simulink model "rician_channel_rectangular"  (R2016b)
settings: Solver=FixedStepAuto  StartTime=0.0  StopTime=2e-6  FixedStep=2*10^(-11)  RelTol=1e-3  EnableMultiTasking=on
libraries: simulink x2, commchan3 x2
settings Model: Creator=MOMENT OF PEACE  LastModifiedBy=MOMENT OF PEACE
settings DataIOCC: LimitDataPoints=on  SaveFormat=Array
settings OptimizationCC: LifeSpan=inf
settings DebuggingCC: SFUnexpectedBacktrackingDiag=warning  SFNoUnconditionalDefaultTransitionDiag=warning  SFExecutionAtInitializationDiag=none
settings HardwareCC: ProdBitPerPointer=32  ProdBitPerSizeT=32  ProdBitPerPtrDiffT=32  ProdLargestAtomicFloat=None  ProdIntDivRoundTo=Undefined  ProdEndianess=Unspecified  ProdWordSize=32  ProdHWDeviceType=32-bit Generic
settings ModelReferenceCC: PropagateSignalLabelsOutOfModel=off
settings GRTTargetCC: TargetLangStandard=C89/C90 (ANSI)  GeneratePreprocessorConditionals=Disable all
settings ConfigComp: CovMetricSettings=dw  CovHtmlReporting=on  CovSaveCumulativeToWorkspaceVar=on  CovSaveSingleToWorkspaceVar=on  CovExternalEMLEnable=off

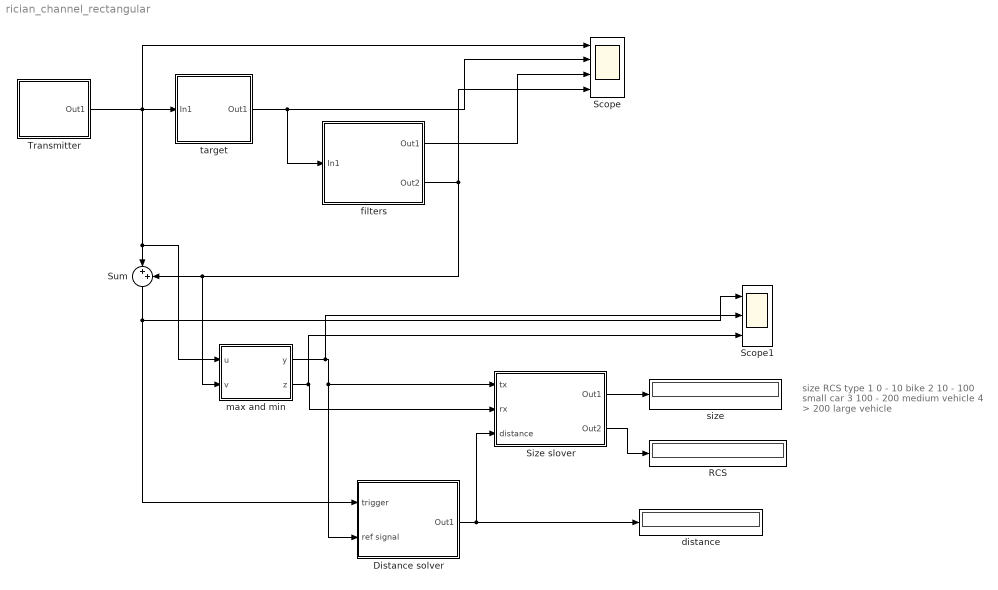
== system rician_channel_rectangular ==
  note: size RCS type
      | 1 0 - 10 bike
      | 2 10 - 100 small car
      | 3 100 - 200 medium vehicle
      | 4 > 200 large vehicle
  Distance solver : Subsystem
  RCS : Display
  Scope : Scope  NumInputPorts=4
  Scope1 : Scope  NumInputPorts=3
  Size slover : Subsystem
  Sum : Sum  Inputs=|++
  Transmitter : Subsystem
  distance : Display
  filters : Subsystem
  max and min : MATLAB Function  TreatAsAtomicUnit=on
  size : Display
  target : Subsystem  mask{d=15, v=30, s=150, snr=5, gain=10}
      mask prompts: d "Distance (m)"; v "Velocity (m/s)"; s "RCS (m^2)"; snr "SNR (dB)"; gain "Gain (dB)"
      mask init:
      | % d denotes the distance and v denotes velocity
      | c = 3e8;    % the speed of light
      | p = 1e-9;   % the width of impulse
      | r = 0.7;    % relectivity
      | rcs = s;
      | w = p * c;
      | 
      | G = 10^(gain/10);       % gain in decimal
      | delay = 2 * d / c;      % phase delay
      | loss = G^2 *  w^2 * rcs/((4 * pi)^3 * d^4);     % path loss
  wires:
  target/1(Out1) -> Scope/2, filters/1(In1)
  filters/1(Out1) -> Scope/3
  filters/2(Out2) -> max and min/2(v), Sum/2, Scope/4
  max and min/2(z) -> Scope1/3, Size slover/2(rx)
  Size slover/1(Out1) -> size/1
  Sum/1 -> Distance solver/1(trigger), Scope1/1
  Distance solver/1(Out1) -> distance/1, Size slover/3(distance)
  Transmitter/1(Out1) -> Scope/1, target/1(In1), max and min/1(u), Sum/1
  Size slover/2(Out2) -> RCS/1
  max and min/1(y) -> Scope1/2, Size slover/1(tx), Distance solver/2(ref signal)

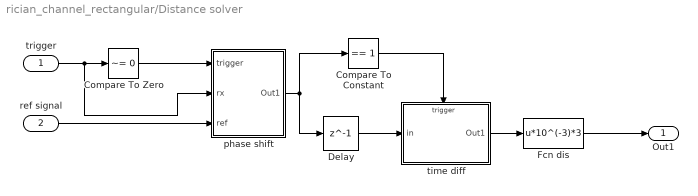
== system rician_channel_rectangular/Distance solver ==
  trigger : Inport
  ref signal : Inport  Port=2
  Compare To Constant : simulink/Logic and Bit Operations/Compare To Constant  relop===  const=1  OutDataTypeStr=boolean
  Compare To Zero : simulink/Logic and Bit Operations/Compare To Zero  relop=~=  OutDataTypeStr=uint8
  Delay : Delay  DelayLength=1  InitialCondition=0
  Fcn dis : Fcn  Expr=u*10^(-3)*3
  phase shift : Subsystem
  time diff : Subsystem  TreatAsAtomicUnit=on
  Out1 : Outport
  wires:
  ref signal/1 -> phase shift/3(ref)
  Fcn dis/1 -> Out1/1
  Compare To Constant/1 -> time diff/Trigger
  trigger/1 -> phase shift/2(rx), Compare To Zero/1
  time diff/1(Out1) -> Fcn dis/1
  Delay/1 -> time diff/1(in)
  phase shift/1(Out1) -> Compare To Constant/1, Delay/1
  Compare To Zero/1 -> phase shift/1(trigger)

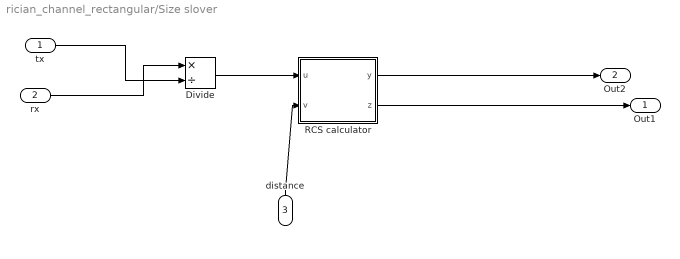
== system rician_channel_rectangular/Size slover ==
  tx : Inport
  rx : Inport  Port=2
  distance : Inport  Port=3
  Divide : Product  Inputs=*/
  RCS calculator : MATLAB Function  TreatAsAtomicUnit=on
  Out1 : Outport
  Out2 : Outport  Port=2
  wires:
  distance/1 -> RCS calculator/2(v)
  tx/1 -> Divide/2
  rx/1 -> Divide/1
  Divide/1 -> RCS calculator/1(u)
  RCS calculator/1(y) -> Out2/1
  RCS calculator/2(z) -> Out1/1

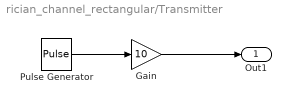
== system rician_channel_rectangular/Transmitter ==
  Gain : Gain  Gain=10
  Pulse Generator : DiscretePulseGenerator  Amplitude=0.004  Period=10000  PulseWidth=50  SampleTime=2e-11
  Out1 : Outport
  wires:
  Gain/1 -> Out1/1
  Pulse Generator/1 -> Gain/1

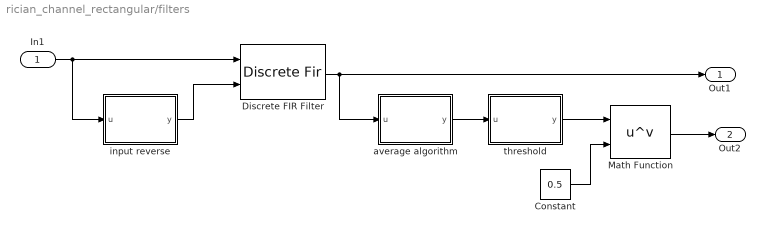
== system rician_channel_rectangular/filters ==
  In1 : Inport
  Constant : Constant  Value=0.5
  Discrete FIR Filter : DiscreteFir  CoefSource=Input port  Coefficients=[1 1 1 1 1 1]  InputProcessing=Columns as channels (frame based)
      settings: InputPortMap=u0,u1
  Math Function : Math  Operator=pow  SaturateOnIntegerOverflow=on
  average algorithm : MATLAB Function  TreatAsAtomicUnit=on
  input reverse : MATLAB Function  TreatAsAtomicUnit=on
  threshold : MATLAB Function  TreatAsAtomicUnit=on
  Out1 : Outport
  Out2 : Outport  Port=2
  wires:
  In1/1 -> Discrete FIR Filter/1, input reverse/1(u)
  average algorithm/1(y) -> threshold/1(u)
  Discrete FIR Filter/1 -> Out1/1, average algorithm/1(u)
  input reverse/1(y) -> Discrete FIR Filter/2
  threshold/1(y) -> Math Function/1
  Math Function/1 -> Out2/1
  Constant/1 -> Math Function/2

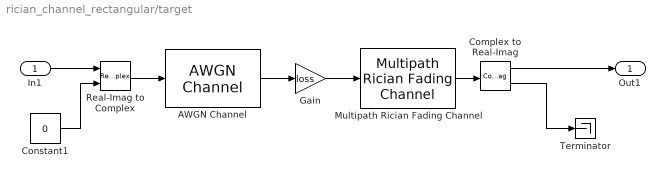
== system rician_channel_rectangular/target ==
  In1 : Inport
  AWGN Channel : commchan3/AWGN Channel  InputProcessing=Columns as channels (frame based)  seed=67  noiseMode="Signal to noise ratio  (SNR)"  EbNodB=10  EsNodB=10  SNRdB=snr  bitsPerSym=1  Ps=0.004/300  Tsym=1  variance=1
  Complex to Real-Imag : ComplexToRealImag
  Constant1 : Constant  Value=0
  Gain : Gain  Gain=loss
  Multipath Rician Fading Channel : commchan3/Multipath Rician Fading Channel  K=100  fdLOS=0  thetaLOS=0  maxDopplerShift=40  spectrumType=Jakes  sigmaGaussian=1/sqrt(2)  coeffRounded=[1 -1.72 0.785]  freqMinMaxRJakes=[0 1]  freqMinMaxAJakes=[0 1]  sigmaGaussian1=1/sqrt(2)  sigmaGaussian2=1/sqrt(2)  centerFreqGaussian1=0  centerFreqGaussian2=0  gainGaussian1=0.5  gainGaussian2=0.5  coeffBell=9  dopplerSpectrum=doppler.jakes  pathDelays=[delay delay+(5e-8) delay+(1e-7)]  avgPathGaindB=[0 -1 -1]  normalizePathGains=on  seed=73  enableProbe=0  openVisAtStart=off  outPathGains=off  outDelay=off
  Real-Imag to Complex : RealImagToComplex
  Terminator : Terminator
  Out1 : Outport
  wires:
  Complex to Real-Imag/1 -> Out1/1
  AWGN Channel/1 -> Gain/1
  Multipath Rician Fading Channel/1 -> Complex to Real-Imag/1
  Constant1/1 -> Real-Imag to Complex/2
  In1/1 -> Real-Imag to Complex/1
  Complex to Real-Imag/2 -> Terminator/1
  Real-Imag to Complex/1 -> AWGN Channel/1
  Gain/1 -> Multipath Rician Fading Channel/1

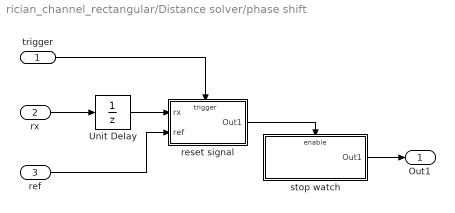
== system rician_channel_rectangular/Distance solver/phase shift ==
  trigger : Inport
  rx : Inport  Port=2
  ref : Inport  Port=3
  Unit Delay : UnitDelay  SampleTime=-1
  reset signal : Subsystem  TreatAsAtomicUnit=on
  stop watch : Subsystem  TreatAsAtomicUnit=on
  Out1 : Outport
  wires:
  reset signal/1(Out1) -> stop watch/Enable
  trigger/1 -> reset signal/Trigger
  stop watch/1(Out1) -> Out1/1
  rx/1 -> Unit Delay/1
  ref/1 -> reset signal/2(ref)
  Unit Delay/1 -> reset signal/1(rx)

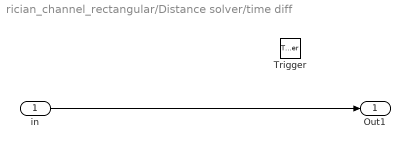
== system rician_channel_rectangular/Distance solver/time diff ==
  in : Inport
  Trigger : TriggerPort  VariantControl=Variant  ZeroCross=off
  Out1 : Outport
  wires:
  in/1 -> Out1/1

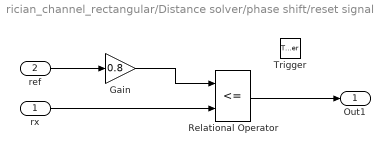
== system rician_channel_rectangular/Distance solver/phase shift/reset signal ==
  rx : Inport
  ref : Inport  Port=2
  Trigger : TriggerPort  TriggerType=falling  VariantControl=Variant
  Gain : Gain  Gain=0.8
  Relational Operator : RelationalOperator  Operator=<=  OutDataTypeStr=boolean  RndMeth=Nearest
  Out1 : Outport
  wires:
  ref/1 -> Gain/1
  Gain/1 -> Relational Operator/1
  rx/1 -> Relational Operator/2
  Relational Operator/1 -> Out1/1

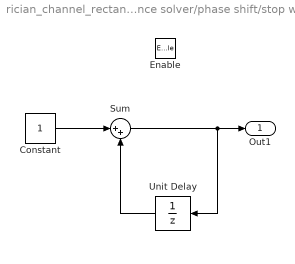
== system rician_channel_rectangular/Distance solver/phase shift/stop watch ==
  Enable : EnablePort  StatesWhenEnabling=reset
  Constant : Constant
  Sum : Sum  Inputs=|++
  Unit Delay : UnitDelay  SampleTime=-1
  Out1 : Outport
  wires:
  Constant/1 -> Sum/1
  Sum/1 -> Unit Delay/1, Out1/1
  Unit Delay/1 -> Sum/2

== matlab function rician_channel_rectangular/filters/average algorithm ==
  data: u input; y output
function y = fcn(u)
%#codegen
persistent summ;
persistent maxm;
n = 200;

if isempty(maxm)
    maxm = -1;
end

if isempty(summ)
    summ = zeros(1,n);
end

if u > max(summ)
    maxm = u;
end

if (u < 0.5*maxm)
    y = 0;
else
    summ = circshift(summ,[0,1]);
    summ(1) = u;
    y = sum(summ) / n;
end

== matlab function rician_channel_rectangular/filters/input reverse ==
  data: u input; y output
function y = fcn(u)
%#codegen

y = u(end:-1:1);

== matlab function rician_channel_rectangular/filters/threshold ==
  data: u input; y output
function y = fcn(u)
%#codegen
persistent maxm;

if isempty(maxm)
    maxm = -1;
end

if u > maxm
    maxm = u;
end

if u > (maxm * 2/3)
    y = u;
else
    y = 0;
end

== matlab function rician_channel_rectangular/max and min ==
  data: u input; y output; v input; z output
function [y,z] = fcn(u,v)
%#codegen
persistent maxm;
persistent minm;

if isempty(maxm)
    maxm = -1;
end

if isempty(minm)
    minm = -1;
end

if u > 0
    maxm = u;
end

if v > 0
    minm = v;
end

y = maxm;
z = minm;

== matlab function rician_channel_rectangular/Size slover/RCS calculator ==
  data: u input; y output; v input; z output
function [y,z] = fcn(u,v)
%#codegen
G = 10;
w = 0.3;
y = 1.69 * u * ((4 * pi)^3 * v^4)/(G^2 *  w^2);
if y < 10
    z = 1;%'bike';
elseif y < 100
    z = 2;%'small car';
elseif y < 200
    z = 3;%'SUV or small truck';
else
    z = 4;%'truck';
end
